simulink model "AM_Mod_Demod"  (R2016a)
settings: Solver=VariableStepAuto  StartTime=0.0  StopTime=1  RelTol=1e-3
settings Model: Creator=Student  LastModifiedBy=Student

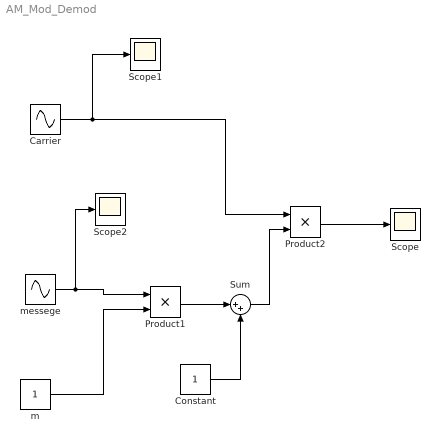
== system AM_Mod_Demod ==
  "Carrier " : Sin  Frequency=2*pi*25  SampleTime=1/5000
  Constant : Constant
  Product1 : Product
  Product2 : Product
  Scope : Scope
  Scope1 : Scope
  Scope2 : Scope
  Sum : Sum  Inputs=|++
  "m " : Constant
  "messege " : Sin  Frequency=2*pi  SampleTime=1/5000
  wires:
  "Carrier "/1 -> Scope1/1, Product2/1
  Sum/1 -> Product2/2
  Product1/1 -> Sum/1
  Constant/1 -> Sum/2
  "m "/1 -> Product1/2
  "messege "/1 -> Scope2/1, Product1/1
  Product2/1 -> Scope/1
